simulink model "SpeedModel"  (R2021a)
settings: Solver=VariableStepAuto  StartTime=0.0  StopTime=1  RelTol=1e-3
values from neighbouring files (symbols this model uses):
  J = moment_of_inertia_after_gear_box    (= 0.002369664)    [Lab_2.m]
  Ke = lsqcurvefit(function_to_cal_voltage, predict_Ke, array_Wnls_speed, voltages')    [Lab_2.m]
  Km = Ke    [Lab_2.m]
  R = resistance    [Lab_2.m]
  U = voltages(i)    [Lab_2.m]
settings Model: Creator=romas  LastModifiedBy=romas

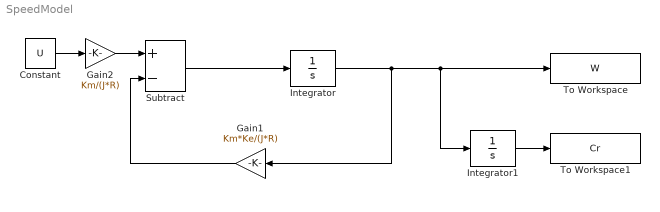
== system SpeedModel ==
  Constant : Constant  Value=U
  Gain1 : Gain  Gain=Km*Ke/(J*R)
  Gain2 : Gain  Gain=Km/(J*R)
  Integrator : Integrator
  Integrator1 : Integrator
  Subtract : Sum  Inputs=+-
  To Workspace : ToWorkspace  VariableName=W  SaveFormat=Timeseries  SampleTime=-1
  To Workspace1 : ToWorkspace  VariableName=Cr  SaveFormat=Timeseries  SampleTime=-1
  wires:
  Constant/1 -> Gain2/1
  Gain1/1 -> Subtract/2
  Subtract/1 -> Integrator/1
  Gain2/1 -> Subtract/1
  Integrator1/1 -> To Workspace1/1
  Integrator/1 -> To Workspace/1, Integrator1/1, Gain1/1
